simulink model "statistics"  (Simulink 7.9)
settings: Solver=FixedStepDiscrete  StartTime=0.0  StopTime=0.0  RelTol=1e-3
libraries: visionstatistics x1, visionconversions x1, visionsources x1
settings Model: Creator=lenovo  LastModifiedBy=lenovo
settings DebuggingCC: SolverPrmCheckMsg=none

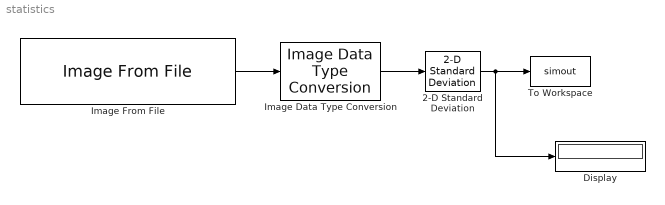
== system statistics ==
  2-D Standard Deviation : visionstatistics/2-D Standard Deviation  run=off  reset_popup=None  directionMode=Entire input  dimension=1  treatSBRowAsCol=on  roiEnable=off  roiType=Rectangles  roiPortion=Entire ROI  roiOutput=Individual statistics for each ROI  roiFlag=off
  Display : Display
  Image Data Type Conversion : visionconversions/Image Data Type Conversion  outDT=double  isSigned=on  wordLen=16  numFracBits=0
  Image From File : visionsources/Image From File  Tag=vipblks_nd  FileName=cameraman.tif  imagePorts=One multidimensional signal  Ts=inf  ImageDataType=Inherit from input image  Signed=on  WordLength=16  sdImageDataType=uint(8)  FractionLengthMode=User-defined  FractionLength=15  OutPortLabels=R|G|B
  To Workspace : ToWorkspace  VariableName=simout  SampleTime=-1  SaveFormat=Timeseries
  wires:
  Image From File/1 -> Image Data Type Conversion/1
  Image Data Type Conversion/1 -> 2-D Standard Deviation/1
  2-D Standard Deviation/1 -> To Workspace/1, Display/1
